simulink model "Zadatak1"  (R2023a)
settings: Solver=VariableStepAuto  StartTime=0.0  StopTime=T_sim  RelTol=1e-3
values from neighbouring files (symbols this model uses):
  Gfden = cell2mat(Gfden)    [Zadatak1_skripta.m]
  Gfnum = cell2mat(Gfnum)    [Zadatak1_skripta.m]
  Ts = 0.01    [Zadatak1_skripta.m]
  w = 1    [Zadatak1_skripta.m]
  Xm = Xm_pom(j)    [Zadatak1_skripta.m]
settings Model: Creator=Acer  LastModifiedBy=Enio
settings SolverCC: AlgebraicLoopSolver=TrustRegion
settings DataIOCC: ReturnWorkspaceOutputs=off
settings DebuggingCC: UnconnectedInputMsg=warning  UnconnectedOutputMsg=warning  UnconnectedLineMsg=warning  ArithmeticOperatorsInVariantConditions=warning
settings ModelReferenceCC: EnableRefExpFcnMdlSchedulingChecks=on
settings SFSimCC: CustomCodeUndefinedFunction=UseInterfaceOnly
settings RTWCC: DLArmComputeVersion=19.05

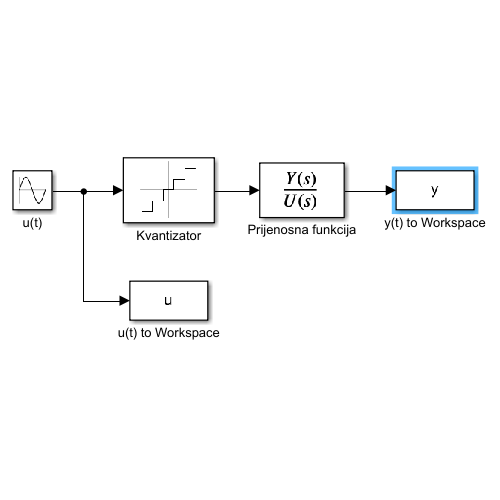
[thumbnail: Simulink's stored preview of the top-level diagram]
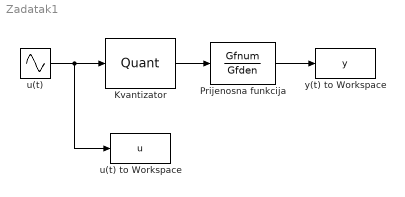
== system Zadatak1 ==
  Kvantizator : Quantizer  QuantizationInterval=D
  Prijenosna funkcija : TransferFcn  Numerator=Gfnum  Denominator=Gfden
  u(t) : Sin  Amplitude=Xm  Frequency=w  SampleTime=0
  u(t) to Workspace : ToWorkspace  VariableName=u  SaveFormat=Timeseries  SampleTime=Ts
  y(t) to Workspace : ToWorkspace  VariableName=y  SaveFormat=Timeseries  SampleTime=Ts
  wires:
  u(t)/1 -> u(t) to Workspace/1, Kvantizator/1
  Kvantizator/1 -> Prijenosna funkcija/1
  Prijenosna funkcija/1 -> y(t) to Workspace/1
